simulink model "Ast_att"  (R2017b)
settings: Solver=ode5  StartTime=0.0  StopTime=2*86400  FixedStep=60  RelTol=1e-3
undefined symbols (not defined in the file): Cube
settings Model: Creator=hazr_sh  LastModifiedBy=hazr_sh

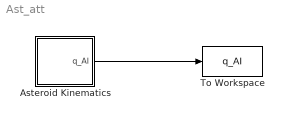
== system Ast_att ==
  Asteroid Kinematics : Subsystem
  To Workspace : ToWorkspace  VariableName=q_AI  SaveFormat=Timeseries  SampleTime=-1
  wires:
  Asteroid Kinematics/1(q_AI) -> To Workspace/1

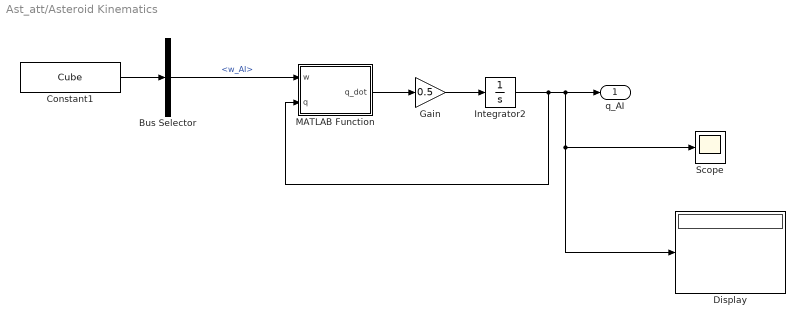
== system Ast_att/Asteroid Kinematics ==
  Bus Selector : BusSelector  OutputSignals=w_AI
  Constant1 : Constant  Value=Cube  VectorParams1D=off  OutDataTypeStr=Bus: slBus1
  Display : Display
  Gain : Gain  Gain=0.5
  Integrator2 : Integrator  InitialCondition=[0 0 0 1]'
  MATLAB Function : MATLAB Function  TreatAsAtomicUnit=on
  Scope : Scope
  q_AI : Outport
  wires:
  MATLAB Function/1(q_dot) -> Gain/1
  Bus Selector/1 -> MATLAB Function/1(w)  "<w_AI>"
  Constant1/1 -> Bus Selector/1
  Gain/1 -> Integrator2/1
  Integrator2/1 -> MATLAB Function/2(q), Display/1, Scope/1, q_AI/1

== matlab function Ast_att/Asteroid Kinematics/MATLAB Function ==
  data: w input; q_dot output; q input
function q_dot = fcn(w,q)

W = [0 w(3) -w(2) w(1)
    -w(3) 0 w(1) w(2)
     w(2) -w(1) 0 w(3)
    -w(1) -w(2) -w(3) 0];

q_dot = W*q;

end
